simulink model "Battery"  (R2018a)
settings: Solver=VariableStepAuto  StartTime=0.0  StopTime=10.0  RelTol=1e-3
model workspace (MAT data in the model file):
  AccessoryLoad = 600
  C_ref = 600
  DrCycles.C505 = [0 1 2 3 4 5 6 7 8 9 10 11 ... (1012 elements, 506x2)]
  DrCycles.FTP = [0 1 2 3 4 5 6 7 8 9 10 11 ... (4956 elements, 2478x2)]
  DrCycles.UDDS = [0 1 2 3 4 5 6 7 8 9 10 11 ... (2746 elements, 1373x2)]
  DrCycles.HWFET = [0 1 2 3 4 5 6 7 8 9 10 11 ... (1532 elements, 766x2)]
  DrCycles.US06 = [0 1 2 3 4 5 6 7 8 9 10 11 ... (1194 elements, 597x2)]
  DrCycles.US06City = [0 1 2 3 4 5 6 7 8 9 10 11 ... (466 elements, 233x2)]
  DrCycles.US06Hwy = [0 1 2 3 4 5 6 7 8 9 10 11 ... (742 elements, 371x2)]
  K = 1.04716227018
  Kc_ref = 0.12
  Ki_ref = 0.01
  Kw_ref = 1.2e-05
  MDL.MotorModel.kc = 0.0452374100719
  MDL.MotorModel.ki = 0.0166666666667
  MDL.MotorModel.kw = 5.06640055941e-05
  MDL.MotorModel.C = 628.29736211
  MDL.MotorModel.MaxTrqOut = 500
  MDL.MotorModel.MaxPwrOut = 100000
  MDL.DrivelineModel.C0 = 600
  MDL.DrivelineModel.C1 = 0.012
  MDL.DrivelineModel.C2 = 4.9e-07
  MDL.DrivelineModel.G = 3.55
  MDL.DrivelineModel.Spinloss = 6
  MDL.DrivelineModel.Ftr_max = 5000
  MDL.DriverModel.Kp = 350
  MDL.DriverModel.Ki = 0
  MDL.DriverModel.Kd = 0
  MDL.DriverModel.BrakeGain = 100
  MDL.DriverModel.Ftr_Max = 5000
  MDL.DriverModel.Ptr_Max = 100000
  MDL.BrakeSys.MaxBrakeForce = 10000
  MDL.BrakeSys.RegenFraction = 0.55
  T_max = 500
  T_ref = 300
  TimeHWFET = 765
  TimeUDDS = 1372
  TimeUS06 = 596
  aeroDragCoeff = 0.38
  airDensity = 1.23
  energyCapacity = 12.6
  frontArea = 2.1
  gravity = 9.81
  inclinationAngle = 0
  inertialMassVeh = 2392
  initialSOC = 0.95
  internalResistance = 0.1
  massVeh = 2300
  openCircuitVoltage = 340
  rollingResistCoeff = 0.01
  w_max = 524
  w_ref = 834
  wheelRadius = 0.34
libraries: simulink x1
settings Model: Creator=100655384  LastModifiedBy=100655384

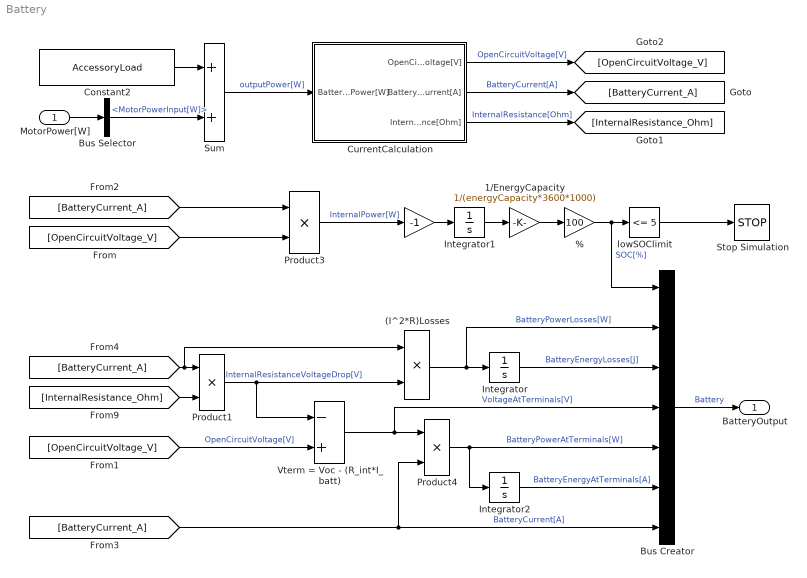
== system Battery ==
  MotorPower[W] : Inport
  " " : Gain  Gain=-1
  % : Gain  Gain=100
  (I^2*R)Losses : Product  RndMeth=Zero
  1/EnergyCapacity : Gain  Gain=1/(energyCapacity*3600*1000)
  Bus Creator : BusCreator  Inputs=7
  Bus Selector : BusSelector  OutputSignals=MotorPowerInput[W]
  Constant2 : Constant  Value=AccessoryLoad
  CurrentCalculation : Subsystem
  Integrator : Integrator  ZeroCross=off
  Integrator1 : Integrator  InitialCondition=energyCapacity*3600*1000*initialSOC  ZeroCross=off
  Integrator2 : Integrator
  Product1 : Product  RndMeth=Zero
  Product3 : Product  RndMeth=Zero
  Product4 : Product  RndMeth=Zero
  Stop Simulation : Stop
  Sum : Sum
  Vterm = Voc - (R_int*I_batt) : Sum  Inputs=-+
  lowSOClimit : simulink/Logic and Bit Operations/Compare To Constant  relop=<=  const=5  OutDataTypeStr=boolean
  BatteryOutput : Outport
  wires:
  CurrentCalculation/2(BatteryCurrent[A]) -> [BatteryCurrent_A]  "BatteryCurrent[A]"
  CurrentCalculation/3(InternalResistance[Ohm]) -> [InternalResistance_Ohm]  "InternalResistance[Ohm]"
  Vterm = Voc - (R_int*I_batt)/1 -> Bus Creator/4, Product4/1  "VoltageAtTerminals[V]"
  [BatteryCurrent_A] -> (I^2*R)Losses/1, Product1/1
  Bus Selector/1 -> Sum/2  "<MotorPowerInput[W]>"
  CurrentCalculation/1(OpenCircuitVoltage[V]) -> [OpenCircuitVoltage_V]  "OpenCircuitVoltage[V]"
  Integrator1/1 -> 1/EnergyCapacity/1
  [InternalResistance_Ohm] -> Product1/2
  " "/1 -> Integrator1/1
  Sum/1 -> CurrentCalculation/1(BatteryPower[W])  "outputPower[W]"
  [BatteryCurrent_A] -> Bus Creator/7, Product4/2  "BatteryCurrent[A]"
  [OpenCircuitVoltage_V] -> Product3/2
  Product1/1 -> (I^2*R)Losses/2, Vterm = Voc - (R_int*I_batt)/1  "InternalResistanceVoltageDrop[V]"
  MotorPower[W]/1 -> Bus Selector/1
  1/EnergyCapacity/1 -> %/1
  Product3/1 -> " "/1  "InternalPower[W]"
  Integrator/1 -> Bus Creator/3  "BatteryEnergyLosses[J]"
  Constant2/1 -> Sum/1
  Product4/1 -> Bus Creator/5, Integrator2/1  "BatteryPowerAtTerminals[W]"
  (I^2*R)Losses/1 -> Bus Creator/2, Integrator/1  "BatteryPowerLosses[W]"
  lowSOClimit/1 -> Stop Simulation/1
  [BatteryCurrent_A] -> Product3/1
  [OpenCircuitVoltage_V] -> Vterm = Voc - (R_int*I_batt)/2  "OpenCircuitVoltage[V]"
  %/1 -> lowSOClimit/1, Bus Creator/1  "SOC[%]"
  Bus Creator/1 -> BatteryOutput/1  "Battery"
  Integrator2/1 -> Bus Creator/6  "BatteryEnergyAtTerminals[A]"

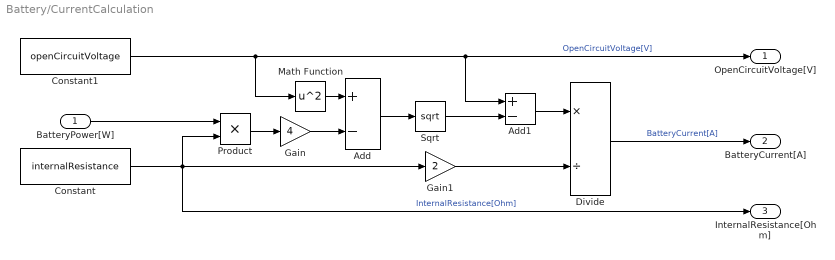
== system Battery/CurrentCalculation ==
  BatteryPower[W] : Inport
  Add : Sum  Inputs=+-
  Add1 : Sum  Inputs=+-
  Constant : Constant  Value=internalResistance
  Constant1 : Constant  Value=openCircuitVoltage
  Divide : Product  Inputs=*/
  Gain : Gain  Gain=4
  Gain1 : Gain  Gain=2
  Math Function : Math  Operator=square  SaturateOnIntegerOverflow=on
  Product : Product  RndMeth=Zero
  Sqrt : Sqrt  SaturateOnIntegerOverflow=on
  OpenCircuitVoltage[V] : Outport
  BatteryCurrent[A] : Outport  Port=2
  InternalResistance[Ohm] : Outport  Port=3
  wires:
  BatteryPower[W]/1 -> Product/1
  Constant/1 -> InternalResistance[Ohm]/1, Gain1/1, Product/2  "InternalResistance[Ohm]"
  Product/1 -> Gain/1
  Constant1/1 -> Math Function/1, OpenCircuitVoltage[V]/1, Add1/1  "OpenCircuitVoltage[V]"
  Math Function/1 -> Add/1
  Gain/1 -> Add/2
  Sqrt/1 -> Add1/2
  Add/1 -> Sqrt/1
  Add1/1 -> Divide/1
  Gain1/1 -> Divide/2
  Divide/1 -> BatteryCurrent[A]/1  "BatteryCurrent[A]"
